simulink model "BSD_RadarInput_SWC"  (R2024a)
settings: Solver=FixedStepDiscrete  StartTime=0.0  StopTime=10.0  FixedStep=0.02  RelTol=1e-3
libraries: simulink x4
settings Model: Creator=pc  LastModifiedBy=pc
settings OptimizationCC: DefaultParameterBehavior=Inlined  EnhancedBackFolding=on  PassReuseOutputArgsAs=Individual arguments  ZeroExternalMemoryAtStartup=off  ZeroInternalMemoryAtStartup=off  OptimizeBlockOrder=speed  DifferentSizesBufferReuse=on  OptimizationCustomize=off  EfficientTunableParamExpr=on
settings DebuggingCC: ParameterTunabilityLossMsg=error
settings SFSimCC: MATLABDynamicMemAlloc=off
settings RTWCC: Description=AUTOSAR  SystemTargetFile=autosar.tlc  GenCodeOnly=on  PackageGeneratedCodeAndArtifacts=on  TemplateMakefile=ert_default_tmf  Toolchain=MinGW64 | CMake/gmake (64-bit Windows)  BuildConfiguration=Release  DataTypeReplacement=CDataTypesFixedWidth  CheckMdlBeforeBuild=Error
settings CodeAppCC: ForceParamTrailComments=on  IgnoreCustomStorageClasses=off  OperatorAnnotations=on  SimulinkDataObjDesc=on  SFDataObjDesc=on  InsertBlockDesc=on
settings STFCustomTargetCC: MultiwordLength=256  ParMdlRefBuildCompliant=on  CompOptLevelCompliant=on  IncludeMdlTerminateFcn=off  CombineOutputUpdateFcns=on  SuppressErrorStatus=on  ERTCustomFileBanners=on  SupportNonFinite=off  SupportComplex=off  SupportContinuousTime=off  SupportNonInlinedSFcns=off  RemoveResetFunc=on  MATLABClassNameForMDSCustomization=Simulink.SoftwareTarget.ERTCustomization  AutosarCompliant=on  GRTInterface=off  LookupTableObjectStructAxisOrder=2,1,3,4,...  LUTObjectStructOrderEvenSpacing=Size,Table,Breakpoints  SystemTargetFile=autosar.tlc
settings ERTTargetCC: TargetLangStandard=C99 (ISO)  ConcurrentExecutionCompliant=off  IncludeMdlTerminateFcn=off  SuppressErrorStatus=on  SupportNonFinite=off  SupportComplex=off  ModelStepFunctionPrototypeControlCompliant=off  CPPClassGenCompliant=off  AutosarCompliant=on  LookupTableObjectStructAxisOrder=2,1,3,4,...  LUTObjectStructOrderEvenSpacing=Size,Table,Breakpoints  InlinedParameterPlacement=NonHierarchical  ERTCustomFileTemplate=example_file_process.tlc  BooleanTrueId=TRUE  BooleanFalseId=FALSE

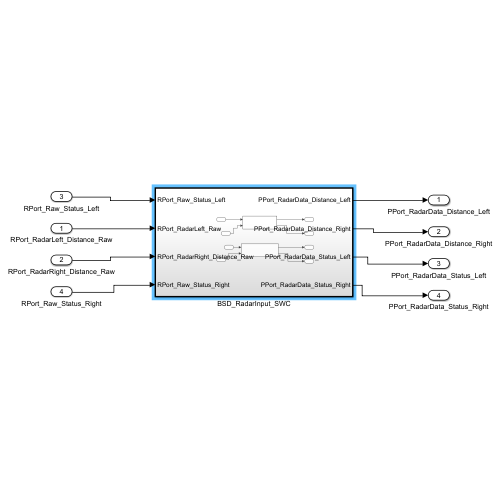
[thumbnail: Simulink's stored preview of the top-level diagram]
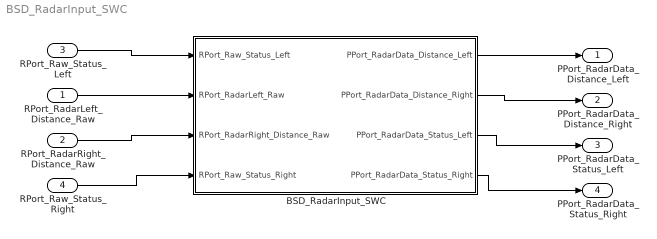
== system BSD_RadarInput_SWC ==
  RPort_RadarLeft_Distance_Raw : Inport  OutDataTypeStr=uint16
  RPort_RadarRight_Distance_Raw : Inport  Port=2  OutDataTypeStr=uint16
  RPort_Raw_Status_Left : Inport  Port=3  OutDataTypeStr=uint8
  RPort_Raw_Status_Right : Inport  Port=4  OutDataTypeStr=uint8
  BSD_RadarInput_SWC : Subsystem  TreatAsAtomicUnit=on  SystemSampleTime=0.02
  PPort_RadarData_Distance_Left : Outport
  PPort_RadarData_Distance_Right : Outport  Port=2
  PPort_RadarData_Status_Left : Outport  Port=3
  PPort_RadarData_Status_Right : Outport  Port=4
  wires:
  RPort_RadarRight_Distance_Raw/1 -> BSD_RadarInput_SWC/3(RPort_RadarRight_Distance_Raw)
  RPort_RadarLeft_Distance_Raw/1 -> BSD_RadarInput_SWC/2(RPort_RadarLeft_Raw)
  RPort_Raw_Status_Left/1 -> BSD_RadarInput_SWC/1(RPort_Raw_Status_Left)
  BSD_RadarInput_SWC/1(PPort_RadarData_Distance_Left) -> PPort_RadarData_Distance_Left/1
  RPort_Raw_Status_Right/1 -> BSD_RadarInput_SWC/4(RPort_Raw_Status_Right)
  BSD_RadarInput_SWC/4(PPort_RadarData_Status_Right) -> PPort_RadarData_Status_Right/1
  BSD_RadarInput_SWC/3(PPort_RadarData_Status_Left) -> PPort_RadarData_Status_Left/1
  BSD_RadarInput_SWC/2(PPort_RadarData_Distance_Right) -> PPort_RadarData_Distance_Right/1

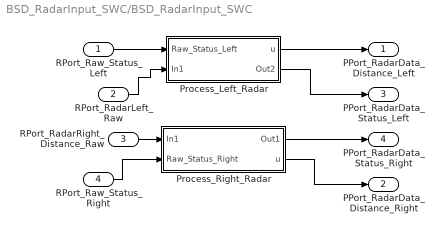
== system BSD_RadarInput_SWC/BSD_RadarInput_SWC ==
  RPort_Raw_Status_Left : Inport
  RPort_RadarLeft_Raw : Inport  Port=2  OutDataTypeStr=uint16
  RPort_RadarRight_Distance_Raw : Inport  Port=3  OutDataTypeStr=uint16
  RPort_Raw_Status_Right : Inport  Port=4
  Process_Left_Radar : Subsystem
  Process_Right_Radar : Subsystem
  PPort_RadarData_Distance_Left : Outport  OutDataTypeStr=single
  PPort_RadarData_Distance_Right : Outport  Port=2  OutDataTypeStr=single
  PPort_RadarData_Status_Left : Outport  Port=3  OutDataTypeStr=uint8
  PPort_RadarData_Status_Right : Outport  Port=4  OutDataTypeStr=uint8
  wires:
  RPort_Raw_Status_Right/1 -> Process_Right_Radar/2(Raw_Status_Right)
  RPort_Raw_Status_Left/1 -> Process_Left_Radar/1(Raw_Status_Left)
  RPort_RadarLeft_Raw/1 -> Process_Left_Radar/2(In1)
  Process_Left_Radar/1(u) -> PPort_RadarData_Distance_Left/1
  RPort_RadarRight_Distance_Raw/1 -> Process_Right_Radar/1(In1)
  Process_Right_Radar/2(u) -> PPort_RadarData_Distance_Right/1
  Process_Left_Radar/2(Out2) -> PPort_RadarData_Status_Left/1
  Process_Right_Radar/1(Out1) -> PPort_RadarData_Status_Right/1

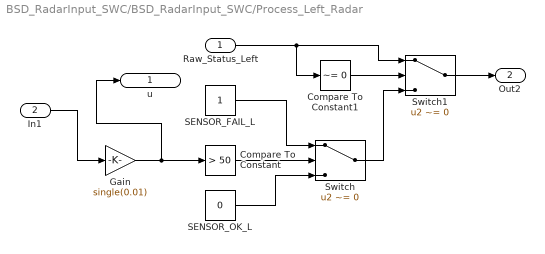
== system BSD_RadarInput_SWC/BSD_RadarInput_SWC/Process_Left_Radar ==
  Raw_Status_Left : Inport
  In1 : Inport  Port=2
  Compare To Constant : simulink/Logic and Bit Operations/Compare To Constant  relop=>  const=50  OutDataTypeStr=uint8
  Compare To Constant1 : simulink/Logic and Bit Operations/Compare To Constant  relop=~=  const=0  OutDataTypeStr=uint8
  Gain : Gain  Gain=single(0.01)  ParamDataTypeStr=single  OutDataTypeStr=single
  SENSOR_FAIL_L : Constant
  SENSOR_OK_L : Constant  Value=0
  Switch : Switch  Criteria=u2 ~= 0  OutDataTypeStr=uint8  SaturateOnIntegerOverflow=off  InputSameDT=off
  Switch1 : Switch  Criteria=u2 ~= 0  Threshold=0.5  SaturateOnIntegerOverflow=off  InputSameDT=off
  u : Outport  OutDataTypeStr=single
  Out2 : Outport  Port=2  OutDataTypeStr=uint8
  wires:
  Switch/1 -> Switch1/3
  In1/1 -> Gain/1
  Gain/1 -> u/1, Compare To Constant/1
  Raw_Status_Left/1 -> Switch1/1, Compare To Constant1/1
  SENSOR_OK_L/1 -> Switch/3
  SENSOR_FAIL_L/1 -> Switch/1
  Compare To Constant/1 -> Switch/2
  Compare To Constant1/1 -> Switch1/2
  Switch1/1 -> Out2/1

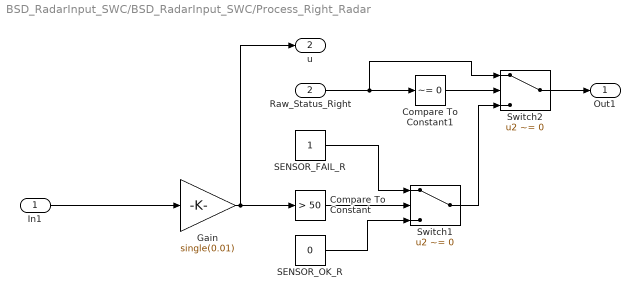
== system BSD_RadarInput_SWC/BSD_RadarInput_SWC/Process_Right_Radar ==
  In1 : Inport
  Raw_Status_Right : Inport  Port=2
  Compare To Constant : simulink/Logic and Bit Operations/Compare To Constant  relop=>  const=50  OutDataTypeStr=uint8
  Compare To Constant1 : simulink/Logic and Bit Operations/Compare To Constant  relop=~=  const=0  OutDataTypeStr=uint8
  Gain : Gain  Gain=single(0.01)  ParamDataTypeStr=single  OutDataTypeStr=single
  SENSOR_FAIL_R : Constant
  SENSOR_OK_R : Constant  Value=0
  Switch1 : Switch  Criteria=u2 ~= 0  OutDataTypeStr=uint8  SaturateOnIntegerOverflow=off  InputSameDT=off
  Switch2 : Switch  Criteria=u2 ~= 0  Threshold=0.5  SaturateOnIntegerOverflow=off  InputSameDT=off
  Out1 : Outport
  u : Outport  Port=2  OutDataTypeStr=single
  wires:
  In1/1 -> Gain/1
  Gain/1 -> u/1, Compare To Constant/1
  Compare To Constant/1 -> Switch1/2
  Compare To Constant1/1 -> Switch2/2
  Raw_Status_Right/1 -> Switch2/1, Compare To Constant1/1
  SENSOR_OK_R/1 -> Switch1/3
  SENSOR_FAIL_R/1 -> Switch1/1
  Switch1/1 -> Switch2/3
  Switch2/1 -> Out1/1
